simulink model "P_PI_PID_2opamp_blocks"  (R2019b)
settings: Solver=VariableStepAuto  StartTime=0.0  StopTime=15  RelTol=1e-3
settings Model: Creator=robom  LastModifiedBy=robom
settings DataIOCC: SaveOutput=off  ReturnWorkspaceOutputs=off
settings DebuggingCC: AlgebraicLoopMsg=none
settings SFSimCC: CustomCodeUndefinedFunction=UseInterfaceOnly

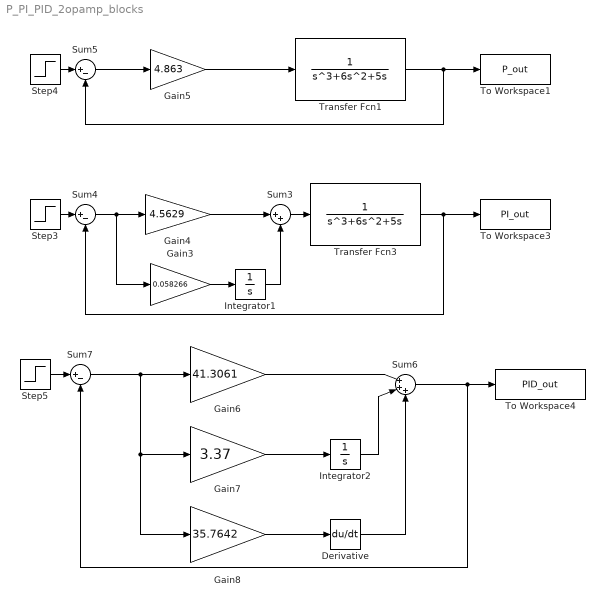
== system P_PI_PID_2opamp_blocks ==
  Derivative : Derivative
  Gain3 : Gain  Gain=0.058266
  Gain4 : Gain  Gain=4.5629
  Gain5 : Gain  Gain=4.863
  Gain6 : Gain  Gain=41.3061
  Gain7 : Gain  Gain=3.37
  Gain8 : Gain  Gain=35.7642
  Integrator1 : Integrator
  Integrator2 : Integrator
  Step3 : Step  Time=0  SampleTime=0
  Step4 : Step  Time=0  SampleTime=0
  Step5 : Step  Time=0  SampleTime=0
  Sum3 : Sum  Inputs=|++
  Sum4 : Sum  Inputs=|+-
  Sum5 : Sum  Inputs=|+-
  Sum6 : Sum  Inputs=|+++
  Sum7 : Sum  Inputs=|+-
  To Workspace1 : ToWorkspace  VariableName=P_out  SampleTime=-1
      settings: Save2DSignal=2-D array (concatenate along first dimension)
  To Workspace3 : ToWorkspace  VariableName=PI_out  SampleTime=-1
      settings: Save2DSignal=2-D array (concatenate along first dimension)
  To Workspace4 : ToWorkspace  VariableName=PID_out  SampleTime=-1
      settings: Save2DSignal=2-D array (concatenate along first dimension)
  Transfer Fcn1 : TransferFcn  Denominator=[1 6 5 0]
  Transfer Fcn3 : TransferFcn  Denominator=[1 6 5 0]
  wires:
  Gain3/1 -> Integrator1/1
  Step3/1 -> Sum4/1
  Integrator1/1 -> Sum3/2
  Sum4/1 -> Gain3/1, Gain4/1
  Gain4/1 -> Sum3/1
  Sum5/1 -> Gain5/1
  Step4/1 -> Sum5/1
  Gain5/1 -> Transfer Fcn1/1
  Sum3/1 -> Transfer Fcn3/1
  Transfer Fcn1/1 -> To Workspace1/1, Sum5/2
  Transfer Fcn3/1 -> To Workspace3/1, Sum4/2
  Gain6/1 -> Sum6/1
  Gain8/1 -> Derivative/1
  Sum6/1 -> To Workspace4/1, Sum7/2
  Integrator2/1 -> Sum6/2
  Sum7/1 -> Gain8/1, Gain7/1, Gain6/1
  Derivative/1 -> Sum6/3
  Gain7/1 -> Integrator2/1
  Step5/1 -> Sum7/1
